simulink model "Constant_TestGen9"  (R2017b)
settings: Solver=FixedStepDiscrete  StartTime=0.0  StopTime=10.0  RelTol=1e-3
undefined symbols (not defined in the file): Block_TestLib, reset
settings Model: Creator=ktrinh  LastModifiedBy=ktrinh
settings DebuggingCC: ParameterOverflowMsg=none

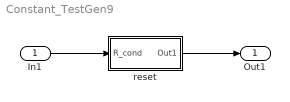
== system Constant_TestGen9 ==
  In1 : Inport
  reset : Subsystem  AncestorBlock=Block_TestLib/reset
  Out1 : Outport
  wires:
  In1/1 -> reset/1(R_cond)
  reset/1(Out1) -> Out1/1

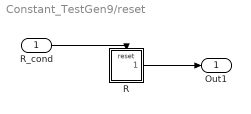
== system Constant_TestGen9/reset ==
  R_cond : Inport  OutDataTypeStr=boolean
  R : Subsystem  TreatAsAtomicUnit=on
  Out1 : Outport
  wires:
  R_cond/1 -> R/Reset
  R/1(Out1) -> Out1/1

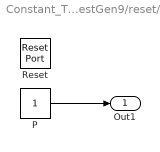
== system Constant_TestGen9/reset/R ==
  Reset : ResetPort  DisableCoverage=on
  P : Constant  VectorParams1D=off  OutDataTypeStr=int32
  Out1 : Outport
  wires:
  P/1 -> Out1/1
